simulink model "magball"  (R2018a)
settings: Solver=VariableStepAuto  StartTime=0.0  StopTime=2.0  RelTol=1e-3
settings Model: Creator=menonpr7  LastModifiedBy=menonpr7

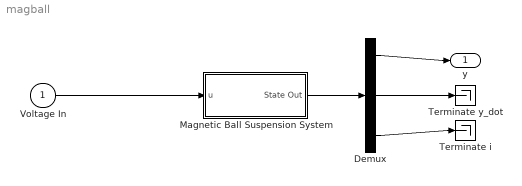
== system magball ==
  Voltage In : Inport
  Demux : Demux  Outputs=3
  Magnetic Ball Suspension System : Subsystem
  Terminate i : Terminator
  Terminate y_dot : Terminator
  "y " : Outport
  wires:
  Voltage In/1 -> Magnetic Ball Suspension System/1(u)
  Magnetic Ball Suspension System/1(State Out) -> Demux/1
  Demux/1 -> "y "/1
  Demux/2 -> Terminate y_dot/1
  Demux/3 -> Terminate i/1

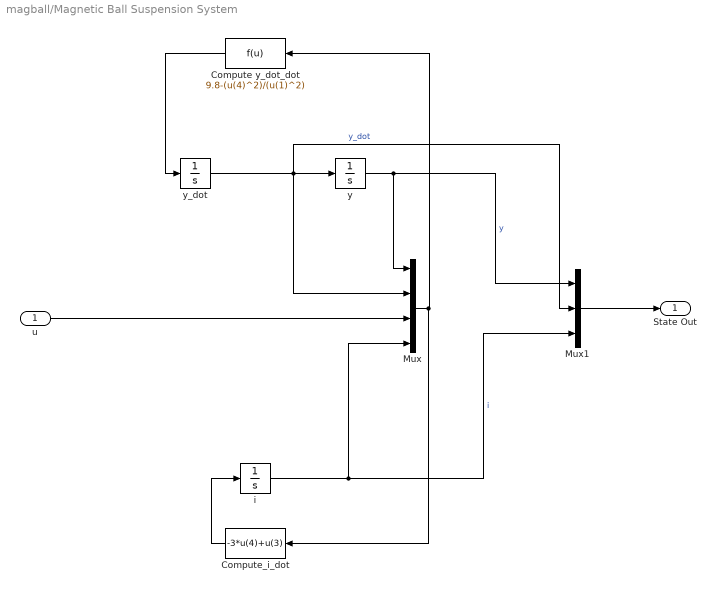
== system magball/Magnetic Ball Suspension System ==
  u : Inport
  Compute y_dot_dot : Fcn  Expr=9.8-(u(4)^2)/(u(1)^2)
  Compute_i_dot : Fcn  Expr=-3*u(4)+u(3)
  Mux : Mux
  Mux1 : Mux  Inputs=3
  i : Integrator
  y : Integrator
  y_dot : Integrator
  State Out : Outport
  wires:
  Compute_i_dot/1 -> i/1
  Compute y_dot_dot/1 -> y_dot/1
  y_dot/1 -> Mux1/2, Mux/2, y/1  "y_dot"
  y/1 -> Mux/1, Mux1/1  "y"
  i/1 -> Mux/4, Mux1/3  "i"
  u/1 -> Mux/3
  Mux/1 -> Compute_i_dot/1, Compute y_dot_dot/1
  Mux1/1 -> State Out/1
